simulink model "cdma7"  (R2012b)
settings: Solver=ode45  StartTime=0.0  StopTime=10.0  RelTol=1e-3
undefined symbols (not defined in the file or in its folder): Fs, get, sided, Two
libraries: dspsnks4 x3, commutil2 x2, commseqgen2 x1, commrandsrc2 x1, dspsigops x1
settings Model: Creator=mcaceres  LastModifiedBy=mcaceres

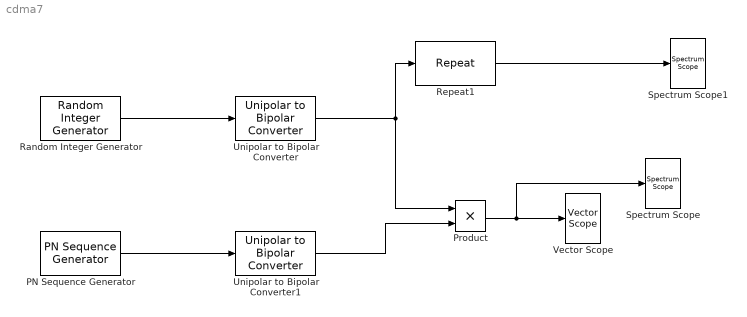
== system cdma7 ==
  PN Sequence Generator : commseqgen2/PN Sequence Generator  poly=[1 1 0 0 0 0 1]  ini_sta=[0 0 0 0 0 1]  outBitMaskSource=Dialog parameter  shift=0  outVarSiz=off  maxOutSizeMode=Dialog parameter  maxOutSize=[10 1]  Ts=(10^-6)/((2^3)-1)  frameBased=off  sampPerFrame=1  reset=off  bitPackedOutputs=off  outDataType=double  numPackedBits=8  bitPackDataSigned=off  bitPackedOutDType=double
  Product : Product  RndMeth=Zero
  Random Integer Generator : commrandsrc2/Random Integer Generator  mul=2  seed=37  Ts=10^-6  frameBased=off  sampPerFrame=1  orient=off  outDataType=double
  Repeat1 : dspsigops/Repeat  N=(2^3)-1  InputProcessing=Columns as channels (frame based)  RateOptions=Allow multirate processing  ic=0  mode=Unused parameter value
  Spectrum Scope : dspsnks4/Spectrum Scope  ScopeProperties=on  Domain=Frequency  HorizSpan=1  UseBuffer=on  BufferSize=128  Overlap=0  TreatMby1Signals=One channel  inpFftLenInherit=on  FFTlength=128  numAvg=20  DisplayProperties=off  AxisGrid=on  Memory=off  FrameNumber=on  AxisLegend=off  AxisZoom=off  OpenScopeAtSimStart=on  OpenScopeImmediately=off  FigPos=get(0,'defaultfigureposition')  AxisProperties=off  XUnits=Hertz  XRange=Two-sided ((-Fs/2...Fs/2])  XDisplay=0  InheritXIncr=on  XIncr=1.0  XLabel=Samples  XLimit=Auto  YUnits=dBW/Hertz  XMax=1  XMin=0  YLabel=Magnitude-squared, dB  LineProperties=off  wintypeSpecScope=Hann  RsSpecScope=50  betaSpecScope=5  winsampSpecScope=Periodic  XAxisParamsVer=6.9  isFrameUpgraded=on
      settings: YMin=-10  YMax=10
  Spectrum Scope1 : dspsnks4/Spectrum Scope  ScopeProperties=on  Domain=Frequency  HorizSpan=1  UseBuffer=on  BufferSize=128  Overlap=0  TreatMby1Signals=One channel  inpFftLenInherit=on  FFTlength=128  numAvg=20  DisplayProperties=off  AxisGrid=on  Memory=off  FrameNumber=on  AxisLegend=off  AxisZoom=off  OpenScopeAtSimStart=on  OpenScopeImmediately=off  FigPos=get(0,'defaultfigureposition')  AxisProperties=off  XUnits=Hertz  XRange=Two-sided ((-Fs/2...Fs/2])  XDisplay=0  InheritXIncr=on  XIncr=1.0  XLabel=Samples  XLimit=Auto  YUnits=dBW/Hertz  XMax=1  XMin=0  YLabel=Magnitude-squared, dB  LineProperties=off  wintypeSpecScope=Hann  RsSpecScope=50  betaSpecScope=5  winsampSpecScope=Periodic  XAxisParamsVer=6.9  isFrameUpgraded=on
      settings: YMin=-10  YMax=10
  Unipolar to Bipolar Converter : commutil2/Unipolar to Bipolar Converter  M=2  polarity=Positive  dataType=Inherit via internal rule
  Unipolar to Bipolar Converter1 : commutil2/Unipolar to Bipolar Converter  M=2  polarity=Positive  dataType=Inherit via internal rule
  Vector Scope : dspsnks4/Vector Scope  ScopeProperties=on  Domain=Time  HorizSpan=3*((2^3)-1)  DisplayProperties=off  AxisGrid=on  Memory=off  FrameNumber=on  AxisLegend=off  AxisZoom=off  OpenScopeAtSimStart=on  OpenScopeImmediately=off  FigPos=get(0,'defaultfigureposition')  AxisProperties=off  XUnits=Hertz  XRange=[0...Fs/2]  InheritXIncr=on  XIncr=1  XLabel=Time  XLimit=Auto  XMin=0  XMax=1  XStart=0  YUnits=dB  YLabel=Amplitude  LineProperties=off  LineStyles=None  LineMarkers=o  XAxisParamsVer=6.9
      settings: YMin=-10  YMax=10
  wires:
  Random Integer Generator/1 -> Unipolar to Bipolar Converter/1
  Unipolar to Bipolar Converter/1 -> Product/1, Repeat1/1
  Unipolar to Bipolar Converter1/1 -> Product/2
  PN Sequence Generator/1 -> Unipolar to Bipolar Converter1/1
  Product/1 -> Spectrum Scope/1, Vector Scope/1
  Repeat1/1 -> Spectrum Scope1/1
